simulink model "Part_e"  (R2016a)
settings: Solver=VariableStepAuto  StartTime=0.0  StopTime=10.0  RelTol=1e-3
values from neighbouring files (symbols this model uses):
  A = [1,0.00958419619475136,0.0104077383156783,0;0,0.880217654134450,2.02956823954280,0;0,-0.102406711940655,0.862350586928406,0;1,0.00958419619475136,0.0104077383156783,1]    [Project_2.m]
  B = [0.0388811995595289;11.5416986681227;10.5268226869341;0.0388811995595289]    [Project_2.m]
  K = place(A,B,[-7,-8,-9,-10])    [Project_2.m]
  Np = 1/N    [Project_2.m]
  x0 = [.2;0;0;0]    [Project_2.m]
settings Model: Creator=ACER  LastModifiedBy=ACER

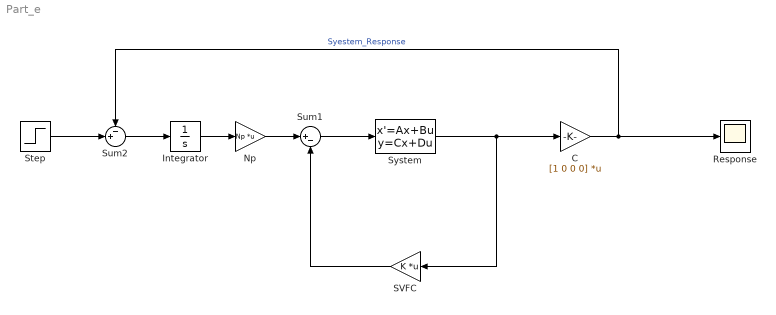
== system Part_e ==
  C : Gain  Gain=[1 0 0 0]  Multiplication=Matrix(K*u)
  Integrator : Integrator
  Np : Gain  Gain=Np  Multiplication=Matrix(K*u)
  Response : Scope
  SVFC : Gain  Gain=K  Multiplication=Matrix(K*u)
  Step : Step  SampleTime=0
  Sum1 : Sum  Inputs=|+-
  Sum2 : Sum  Inputs=-+|
  System : StateSpace  A=A  B=B  C=eye(4)  D=[0;0;0;0]  X0=x0
  wires:
  Sum1/1 -> System/1
  Integrator/1 -> Np/1
  Sum2/1 -> Integrator/1
  Np/1 -> Sum1/1
  SVFC/1 -> Sum1/2
  C/1 -> Sum2/1, Response/1  "Syestem_Response"
  System/1 -> C/1, SVFC/1
  Step/1 -> Sum2/2
